simulink model "TrajectoryGenerator3DOF"  (R2023b)
settings: Solver=FixedStepDiscrete  StartTime=0.0  StopTime=1.364*1.4  FixedStep=0.002  RelTol=1e-3
undefined symbols (not defined in the file or in its folder): M_z, Smoothers, Ts
(part 3 of 4)

== system TrajectoryGenerator3DOF/Trajectory Generator17/M22 ==
  x : Inport
  Discrete FIR Filter1 : DiscreteFir  Coefficients=1/N/Ts*[1 zeros(1,N-1) -1]  InitialStates=Q0  SampleTime=Ts
  Discrete Filter : DiscreteFilter  Numerator=[0 Ts]  Denominator=[1 -1]  InitialStates=Q0  SampleTime=Ts
  y : Outport
  dy : Outport  Port=2
  wires:
  Discrete FIR Filter1/1 -> Discrete Filter/1, dy/1
  x/1 -> Discrete FIR Filter1/1
  Discrete Filter/1 -> y/1

== system TrajectoryGenerator3DOF/Trajectory Generator17/M23 ==
  x : Inport
  Discrete FIR Filter1 : DiscreteFir  Coefficients=1/N/Ts*[1 zeros(1,N-1) -1]  InitialStates=Q0  SampleTime=Ts
  Discrete Filter : DiscreteFilter  Numerator=[0 Ts]  Denominator=[1 -1]  InitialStates=Q0  SampleTime=Ts
  y : Outport
  dy : Outport  Port=2
  wires:
  Discrete FIR Filter1/1 -> Discrete Filter/1, dy/1
  x/1 -> Discrete FIR Filter1/1
  Discrete Filter/1 -> y/1

== system TrajectoryGenerator3DOF/Trajectory Generator17/M24 ==
  x : Inport
  Discrete FIR Filter1 : DiscreteFir  Coefficients=1/N/Ts*[1 zeros(1,N-1) -1]  InitialStates=Q0  SampleTime=Ts
  Discrete Filter : DiscreteFilter  Numerator=[0 Ts]  Denominator=[1 -1]  InitialStates=Q0  SampleTime=Ts
  y : Outport
  dy : Outport  Port=2
  wires:
  Discrete FIR Filter1/1 -> Discrete Filter/1, dy/1
  x/1 -> Discrete FIR Filter1/1
  Discrete Filter/1 -> y/1

== system TrajectoryGenerator3DOF/Trajectory Generator17/M33 ==
  x : Inport
  Discrete FIR Filter1 : DiscreteFir  Coefficients=1/N/Ts*[1 zeros(1,N-1) -1]  InitialStates=Q0  SampleTime=Ts
  Discrete Filter : DiscreteFilter  Numerator=[0 Ts]  Denominator=[1 -1]  InitialStates=Q0  SampleTime=Ts
  y : Outport
  dy : Outport  Port=2
  wires:
  Discrete FIR Filter1/1 -> Discrete Filter/1, dy/1
  x/1 -> Discrete FIR Filter1/1
  Discrete Filter/1 -> y/1

== system TrajectoryGenerator3DOF/Trajectory Generator17/M34 ==
  x : Inport
  Discrete FIR Filter1 : DiscreteFir  Coefficients=1/N/Ts*[1 zeros(1,N-1) -1]  InitialStates=Q0  SampleTime=Ts
  Discrete Filter : DiscreteFilter  Numerator=[0 Ts]  Denominator=[1 -1]  InitialStates=Q0  SampleTime=Ts
  y : Outport
  dy : Outport  Port=2
  wires:
  Discrete FIR Filter1/1 -> Discrete Filter/1, dy/1
  x/1 -> Discrete FIR Filter1/1
  Discrete Filter/1 -> y/1

== system TrajectoryGenerator3DOF/Trajectory Generator17/M44 ==
  x : Inport
  Discrete FIR Filter1 : DiscreteFir  Coefficients=1/N/Ts*[1 zeros(1,N-1) -1]  InitialStates=Q0  SampleTime=Ts
  Discrete Filter : DiscreteFilter  Numerator=[0 Ts]  Denominator=[1 -1]  InitialStates=Q0  SampleTime=Ts
  y : Outport
  dy : Outport  Port=2
  wires:
  Discrete FIR Filter1/1 -> Discrete Filter/1, dy/1
  x/1 -> Discrete FIR Filter1/1
  Discrete Filter/1 -> y/1

== system TrajectoryGenerator3DOF/Trajectory Generator18/M11 ==
  x : Inport
  Discrete FIR Filter1 : DiscreteFir  Coefficients=1/N/Ts*[1 zeros(1,N-1) -1]  InitialStates=Q0  SampleTime=Ts
  Discrete Filter : DiscreteFilter  Numerator=[0 Ts]  Denominator=[1 -1]  InitialStates=Q0  SampleTime=Ts
  y : Outport
  dy : Outport  Port=2
  wires:
  Discrete FIR Filter1/1 -> Discrete Filter/1, dy/1
  x/1 -> Discrete FIR Filter1/1
  Discrete Filter/1 -> y/1

== system TrajectoryGenerator3DOF/Trajectory Generator18/M12 ==
  x : Inport
  Discrete FIR Filter1 : DiscreteFir  Coefficients=1/N/Ts*[1 zeros(1,N-1) -1]  InitialStates=Q0  SampleTime=Ts
  Discrete Filter : DiscreteFilter  Numerator=[0 Ts]  Denominator=[1 -1]  InitialStates=Q0  SampleTime=Ts
  y : Outport
  dy : Outport  Port=2
  wires:
  Discrete FIR Filter1/1 -> Discrete Filter/1, dy/1
  x/1 -> Discrete FIR Filter1/1
  Discrete Filter/1 -> y/1

== system TrajectoryGenerator3DOF/Trajectory Generator18/M13 ==
  x : Inport
  Discrete FIR Filter1 : DiscreteFir  Coefficients=1/N/Ts*[1 zeros(1,N-1) -1]  InitialStates=Q0  SampleTime=Ts
  Discrete Filter : DiscreteFilter  Numerator=[0 Ts]  Denominator=[1 -1]  InitialStates=Q0  SampleTime=Ts
  y : Outport
  dy : Outport  Port=2
  wires:
  Discrete FIR Filter1/1 -> Discrete Filter/1, dy/1
  x/1 -> Discrete FIR Filter1/1
  Discrete Filter/1 -> y/1

== system TrajectoryGenerator3DOF/Trajectory Generator18/M14 ==
  x : Inport
  Discrete FIR Filter1 : DiscreteFir  Coefficients=1/N/Ts*[1 zeros(1,N-1) -1]  InitialStates=Q0  SampleTime=Ts
  Discrete Filter : DiscreteFilter  Numerator=[0 Ts]  Denominator=[1 -1]  InitialStates=Q0  SampleTime=Ts
  y : Outport
  dy : Outport  Port=2
  wires:
  Discrete FIR Filter1/1 -> Discrete Filter/1, dy/1
  x/1 -> Discrete FIR Filter1/1
  Discrete Filter/1 -> y/1

== system TrajectoryGenerator3DOF/Trajectory Generator18/M22 ==
  x : Inport
  Discrete FIR Filter1 : DiscreteFir  Coefficients=1/N/Ts*[1 zeros(1,N-1) -1]  InitialStates=Q0  SampleTime=Ts
  Discrete Filter : DiscreteFilter  Numerator=[0 Ts]  Denominator=[1 -1]  InitialStates=Q0  SampleTime=Ts
  y : Outport
  dy : Outport  Port=2
  wires:
  Discrete FIR Filter1/1 -> Discrete Filter/1, dy/1
  x/1 -> Discrete FIR Filter1/1
  Discrete Filter/1 -> y/1

== system TrajectoryGenerator3DOF/Trajectory Generator18/M23 ==
  x : Inport
  Discrete FIR Filter1 : DiscreteFir  Coefficients=1/N/Ts*[1 zeros(1,N-1) -1]  InitialStates=Q0  SampleTime=Ts
  Discrete Filter : DiscreteFilter  Numerator=[0 Ts]  Denominator=[1 -1]  InitialStates=Q0  SampleTime=Ts
  y : Outport
  dy : Outport  Port=2
  wires:
  Discrete FIR Filter1/1 -> Discrete Filter/1, dy/1
  x/1 -> Discrete FIR Filter1/1
  Discrete Filter/1 -> y/1

== system TrajectoryGenerator3DOF/Trajectory Generator18/M24 ==
  x : Inport
  Discrete FIR Filter1 : DiscreteFir  Coefficients=1/N/Ts*[1 zeros(1,N-1) -1]  InitialStates=Q0  SampleTime=Ts
  Discrete Filter : DiscreteFilter  Numerator=[0 Ts]  Denominator=[1 -1]  InitialStates=Q0  SampleTime=Ts
  y : Outport
  dy : Outport  Port=2
  wires:
  Discrete FIR Filter1/1 -> Discrete Filter/1, dy/1
  x/1 -> Discrete FIR Filter1/1
  Discrete Filter/1 -> y/1

== system TrajectoryGenerator3DOF/Trajectory Generator18/M33 ==
  x : Inport
  Discrete FIR Filter1 : DiscreteFir  Coefficients=1/N/Ts*[1 zeros(1,N-1) -1]  InitialStates=Q0  SampleTime=Ts
  Discrete Filter : DiscreteFilter  Numerator=[0 Ts]  Denominator=[1 -1]  InitialStates=Q0  SampleTime=Ts
  y : Outport
  dy : Outport  Port=2
  wires:
  Discrete FIR Filter1/1 -> Discrete Filter/1, dy/1
  x/1 -> Discrete FIR Filter1/1
  Discrete Filter/1 -> y/1

== system TrajectoryGenerator3DOF/Trajectory Generator18/M34 ==
  x : Inport
  Discrete FIR Filter1 : DiscreteFir  Coefficients=1/N/Ts*[1 zeros(1,N-1) -1]  InitialStates=Q0  SampleTime=Ts
  Discrete Filter : DiscreteFilter  Numerator=[0 Ts]  Denominator=[1 -1]  InitialStates=Q0  SampleTime=Ts
  y : Outport
  dy : Outport  Port=2
  wires:
  Discrete FIR Filter1/1 -> Discrete Filter/1, dy/1
  x/1 -> Discrete FIR Filter1/1
  Discrete Filter/1 -> y/1

== system TrajectoryGenerator3DOF/Trajectory Generator18/M44 ==
  x : Inport
  Discrete FIR Filter1 : DiscreteFir  Coefficients=1/N/Ts*[1 zeros(1,N-1) -1]  InitialStates=Q0  SampleTime=Ts
  Discrete Filter : DiscreteFilter  Numerator=[0 Ts]  Denominator=[1 -1]  InitialStates=Q0  SampleTime=Ts
  y : Outport
  dy : Outport  Port=2
  wires:
  Discrete FIR Filter1/1 -> Discrete Filter/1, dy/1
  x/1 -> Discrete FIR Filter1/1
  Discrete Filter/1 -> y/1

== system TrajectoryGenerator3DOF/Trajectory Generator19/M11 ==
  x : Inport
  Discrete FIR Filter1 : DiscreteFir  Coefficients=1/N/Ts*[1 zeros(1,N-1) -1]  InitialStates=Q0  SampleTime=Ts
  Discrete Filter : DiscreteFilter  Numerator=[0 Ts]  Denominator=[1 -1]  InitialStates=Q0  SampleTime=Ts
  y : Outport
  dy : Outport  Port=2
  wires:
  Discrete FIR Filter1/1 -> Discrete Filter/1, dy/1
  x/1 -> Discrete FIR Filter1/1
  Discrete Filter/1 -> y/1

== system TrajectoryGenerator3DOF/Trajectory Generator19/M12 ==
  x : Inport
  Discrete FIR Filter1 : DiscreteFir  Coefficients=1/N/Ts*[1 zeros(1,N-1) -1]  InitialStates=Q0  SampleTime=Ts
  Discrete Filter : DiscreteFilter  Numerator=[0 Ts]  Denominator=[1 -1]  InitialStates=Q0  SampleTime=Ts
  y : Outport
  dy : Outport  Port=2
  wires:
  Discrete FIR Filter1/1 -> Discrete Filter/1, dy/1
  x/1 -> Discrete FIR Filter1/1
  Discrete Filter/1 -> y/1

== system TrajectoryGenerator3DOF/Trajectory Generator19/M13 ==
  x : Inport
  Discrete FIR Filter1 : DiscreteFir  Coefficients=1/N/Ts*[1 zeros(1,N-1) -1]  InitialStates=Q0  SampleTime=Ts
  Discrete Filter : DiscreteFilter  Numerator=[0 Ts]  Denominator=[1 -1]  InitialStates=Q0  SampleTime=Ts
  y : Outport
  dy : Outport  Port=2
  wires:
  Discrete FIR Filter1/1 -> Discrete Filter/1, dy/1
  x/1 -> Discrete FIR Filter1/1
  Discrete Filter/1 -> y/1

== system TrajectoryGenerator3DOF/Trajectory Generator19/M14 ==
  x : Inport
  Discrete FIR Filter1 : DiscreteFir  Coefficients=1/N/Ts*[1 zeros(1,N-1) -1]  InitialStates=Q0  SampleTime=Ts
  Discrete Filter : DiscreteFilter  Numerator=[0 Ts]  Denominator=[1 -1]  InitialStates=Q0  SampleTime=Ts
  y : Outport
  dy : Outport  Port=2
  wires:
  Discrete FIR Filter1/1 -> Discrete Filter/1, dy/1
  x/1 -> Discrete FIR Filter1/1
  Discrete Filter/1 -> y/1

== system TrajectoryGenerator3DOF/Trajectory Generator19/M22 ==
  x : Inport
  Discrete FIR Filter1 : DiscreteFir  Coefficients=1/N/Ts*[1 zeros(1,N-1) -1]  InitialStates=Q0  SampleTime=Ts
  Discrete Filter : DiscreteFilter  Numerator=[0 Ts]  Denominator=[1 -1]  InitialStates=Q0  SampleTime=Ts
  y : Outport
  dy : Outport  Port=2
  wires:
  Discrete FIR Filter1/1 -> Discrete Filter/1, dy/1
  x/1 -> Discrete FIR Filter1/1
  Discrete Filter/1 -> y/1

== system TrajectoryGenerator3DOF/Trajectory Generator19/M23 ==
  x : Inport
  Discrete FIR Filter1 : DiscreteFir  Coefficients=1/N/Ts*[1 zeros(1,N-1) -1]  InitialStates=Q0  SampleTime=Ts
  Discrete Filter : DiscreteFilter  Numerator=[0 Ts]  Denominator=[1 -1]  InitialStates=Q0  SampleTime=Ts
  y : Outport
  dy : Outport  Port=2
  wires:
  Discrete FIR Filter1/1 -> Discrete Filter/1, dy/1
  x/1 -> Discrete FIR Filter1/1
  Discrete Filter/1 -> y/1

== system TrajectoryGenerator3DOF/Trajectory Generator19/M24 ==
  x : Inport
  Discrete FIR Filter1 : DiscreteFir  Coefficients=1/N/Ts*[1 zeros(1,N-1) -1]  InitialStates=Q0  SampleTime=Ts
  Discrete Filter : DiscreteFilter  Numerator=[0 Ts]  Denominator=[1 -1]  InitialStates=Q0  SampleTime=Ts
  y : Outport
  dy : Outport  Port=2
  wires:
  Discrete FIR Filter1/1 -> Discrete Filter/1, dy/1
  x/1 -> Discrete FIR Filter1/1
  Discrete Filter/1 -> y/1

== system TrajectoryGenerator3DOF/Trajectory Generator19/M33 ==
  x : Inport
  Discrete FIR Filter1 : DiscreteFir  Coefficients=1/N/Ts*[1 zeros(1,N-1) -1]  InitialStates=Q0  SampleTime=Ts
  Discrete Filter : DiscreteFilter  Numerator=[0 Ts]  Denominator=[1 -1]  InitialStates=Q0  SampleTime=Ts
  y : Outport
  dy : Outport  Port=2
  wires:
  Discrete FIR Filter1/1 -> Discrete Filter/1, dy/1
  x/1 -> Discrete FIR Filter1/1
  Discrete Filter/1 -> y/1

== system TrajectoryGenerator3DOF/Trajectory Generator19/M34 ==
  x : Inport
  Discrete FIR Filter1 : DiscreteFir  Coefficients=1/N/Ts*[1 zeros(1,N-1) -1]  InitialStates=Q0  SampleTime=Ts
  Discrete Filter : DiscreteFilter  Numerator=[0 Ts]  Denominator=[1 -1]  InitialStates=Q0  SampleTime=Ts
  y : Outport
  dy : Outport  Port=2
  wires:
  Discrete FIR Filter1/1 -> Discrete Filter/1, dy/1
  x/1 -> Discrete FIR Filter1/1
  Discrete Filter/1 -> y/1

== system TrajectoryGenerator3DOF/Trajectory Generator19/M44 ==
  x : Inport
  Discrete FIR Filter1 : DiscreteFir  Coefficients=1/N/Ts*[1 zeros(1,N-1) -1]  InitialStates=Q0  SampleTime=Ts
  Discrete Filter : DiscreteFilter  Numerator=[0 Ts]  Denominator=[1 -1]  InitialStates=Q0  SampleTime=Ts
  y : Outport
  dy : Outport  Port=2
  wires:
  Discrete FIR Filter1/1 -> Discrete Filter/1, dy/1
  x/1 -> Discrete FIR Filter1/1
  Discrete Filter/1 -> y/1

== system TrajectoryGenerator3DOF/Trajectory Generator2/M11 ==
  x : Inport
  Discrete FIR Filter1 : DiscreteFir  Coefficients=1/N/Ts*[1 zeros(1,N-1) -1]  InitialStates=Q0  SampleTime=Ts
  Discrete Filter : DiscreteFilter  Numerator=[0 Ts]  Denominator=[1 -1]  InitialStates=Q0  SampleTime=Ts
  y : Outport
  dy : Outport  Port=2
  wires:
  Discrete FIR Filter1/1 -> Discrete Filter/1, dy/1
  x/1 -> Discrete FIR Filter1/1
  Discrete Filter/1 -> y/1

== system TrajectoryGenerator3DOF/Trajectory Generator2/M12 ==
  x : Inport
  Discrete FIR Filter1 : DiscreteFir  Coefficients=1/N/Ts*[1 zeros(1,N-1) -1]  InitialStates=Q0  SampleTime=Ts
  Discrete Filter : DiscreteFilter  Numerator=[0 Ts]  Denominator=[1 -1]  InitialStates=Q0  SampleTime=Ts
  y : Outport
  dy : Outport  Port=2
  wires:
  Discrete FIR Filter1/1 -> Discrete Filter/1, dy/1
  x/1 -> Discrete FIR Filter1/1
  Discrete Filter/1 -> y/1

== system TrajectoryGenerator3DOF/Trajectory Generator2/M13 ==
  x : Inport
  Discrete FIR Filter1 : DiscreteFir  Coefficients=1/N/Ts*[1 zeros(1,N-1) -1]  InitialStates=Q0  SampleTime=Ts
  Discrete Filter : DiscreteFilter  Numerator=[0 Ts]  Denominator=[1 -1]  InitialStates=Q0  SampleTime=Ts
  y : Outport
  dy : Outport  Port=2
  wires:
  Discrete FIR Filter1/1 -> Discrete Filter/1, dy/1
  x/1 -> Discrete FIR Filter1/1
  Discrete Filter/1 -> y/1

== system TrajectoryGenerator3DOF/Trajectory Generator2/M14 ==
  x : Inport
  Discrete FIR Filter1 : DiscreteFir  Coefficients=1/N/Ts*[1 zeros(1,N-1) -1]  InitialStates=Q0  SampleTime=Ts
  Discrete Filter : DiscreteFilter  Numerator=[0 Ts]  Denominator=[1 -1]  InitialStates=Q0  SampleTime=Ts
  y : Outport
  dy : Outport  Port=2
  wires:
  Discrete FIR Filter1/1 -> Discrete Filter/1, dy/1
  x/1 -> Discrete FIR Filter1/1
  Discrete Filter/1 -> y/1

== system TrajectoryGenerator3DOF/Trajectory Generator2/M22 ==
  x : Inport
  Discrete FIR Filter1 : DiscreteFir  Coefficients=1/N/Ts*[1 zeros(1,N-1) -1]  InitialStates=Q0  SampleTime=Ts
  Discrete Filter : DiscreteFilter  Numerator=[0 Ts]  Denominator=[1 -1]  InitialStates=Q0  SampleTime=Ts
  y : Outport
  dy : Outport  Port=2
  wires:
  Discrete FIR Filter1/1 -> Discrete Filter/1, dy/1
  x/1 -> Discrete FIR Filter1/1
  Discrete Filter/1 -> y/1

== system TrajectoryGenerator3DOF/Trajectory Generator2/M23 ==
  x : Inport
  Discrete FIR Filter1 : DiscreteFir  Coefficients=1/N/Ts*[1 zeros(1,N-1) -1]  InitialStates=Q0  SampleTime=Ts
  Discrete Filter : DiscreteFilter  Numerator=[0 Ts]  Denominator=[1 -1]  InitialStates=Q0  SampleTime=Ts
  y : Outport
  dy : Outport  Port=2
  wires:
  Discrete FIR Filter1/1 -> Discrete Filter/1, dy/1
  x/1 -> Discrete FIR Filter1/1
  Discrete Filter/1 -> y/1

== system TrajectoryGenerator3DOF/Trajectory Generator2/M24 ==
  x : Inport
  Discrete FIR Filter1 : DiscreteFir  Coefficients=1/N/Ts*[1 zeros(1,N-1) -1]  InitialStates=Q0  SampleTime=Ts
  Discrete Filter : DiscreteFilter  Numerator=[0 Ts]  Denominator=[1 -1]  InitialStates=Q0  SampleTime=Ts
  y : Outport
  dy : Outport  Port=2
  wires:
  Discrete FIR Filter1/1 -> Discrete Filter/1, dy/1
  x/1 -> Discrete FIR Filter1/1
  Discrete Filter/1 -> y/1

== system TrajectoryGenerator3DOF/Trajectory Generator2/M33 ==
  x : Inport
  Discrete FIR Filter1 : DiscreteFir  Coefficients=1/N/Ts*[1 zeros(1,N-1) -1]  InitialStates=Q0  SampleTime=Ts
  Discrete Filter : DiscreteFilter  Numerator=[0 Ts]  Denominator=[1 -1]  InitialStates=Q0  SampleTime=Ts
  y : Outport
  dy : Outport  Port=2
  wires:
  Discrete FIR Filter1/1 -> Discrete Filter/1, dy/1
  x/1 -> Discrete FIR Filter1/1
  Discrete Filter/1 -> y/1

== system TrajectoryGenerator3DOF/Trajectory Generator2/M34 ==
  x : Inport
  Discrete FIR Filter1 : DiscreteFir  Coefficients=1/N/Ts*[1 zeros(1,N-1) -1]  InitialStates=Q0  SampleTime=Ts
  Discrete Filter : DiscreteFilter  Numerator=[0 Ts]  Denominator=[1 -1]  InitialStates=Q0  SampleTime=Ts
  y : Outport
  dy : Outport  Port=2
  wires:
  Discrete FIR Filter1/1 -> Discrete Filter/1, dy/1
  x/1 -> Discrete FIR Filter1/1
  Discrete Filter/1 -> y/1

== system TrajectoryGenerator3DOF/Trajectory Generator2/M44 ==
  x : Inport
  Discrete FIR Filter1 : DiscreteFir  Coefficients=1/N/Ts*[1 zeros(1,N-1) -1]  InitialStates=Q0  SampleTime=Ts
  Discrete Filter : DiscreteFilter  Numerator=[0 Ts]  Denominator=[1 -1]  InitialStates=Q0  SampleTime=Ts
  y : Outport
  dy : Outport  Port=2
  wires:
  Discrete FIR Filter1/1 -> Discrete Filter/1, dy/1
  x/1 -> Discrete FIR Filter1/1
  Discrete Filter/1 -> y/1

== system TrajectoryGenerator3DOF/Trajectory Generator20/M11 ==
  x : Inport
  Discrete FIR Filter1 : DiscreteFir  Coefficients=1/N/Ts*[1 zeros(1,N-1) -1]  InitialStates=Q0  SampleTime=Ts
  Discrete Filter : DiscreteFilter  Numerator=[0 Ts]  Denominator=[1 -1]  InitialStates=Q0  SampleTime=Ts
  y : Outport
  dy : Outport  Port=2
  wires:
  Discrete FIR Filter1/1 -> Discrete Filter/1, dy/1
  x/1 -> Discrete FIR Filter1/1
  Discrete Filter/1 -> y/1

== system TrajectoryGenerator3DOF/Trajectory Generator20/M12 ==
  x : Inport
  Discrete FIR Filter1 : DiscreteFir  Coefficients=1/N/Ts*[1 zeros(1,N-1) -1]  InitialStates=Q0  SampleTime=Ts
  Discrete Filter : DiscreteFilter  Numerator=[0 Ts]  Denominator=[1 -1]  InitialStates=Q0  SampleTime=Ts
  y : Outport
  dy : Outport  Port=2
  wires:
  Discrete FIR Filter1/1 -> Discrete Filter/1, dy/1
  x/1 -> Discrete FIR Filter1/1
  Discrete Filter/1 -> y/1

== system TrajectoryGenerator3DOF/Trajectory Generator20/M13 ==
  x : Inport
  Discrete FIR Filter1 : DiscreteFir  Coefficients=1/N/Ts*[1 zeros(1,N-1) -1]  InitialStates=Q0  SampleTime=Ts
  Discrete Filter : DiscreteFilter  Numerator=[0 Ts]  Denominator=[1 -1]  InitialStates=Q0  SampleTime=Ts
  y : Outport
  dy : Outport  Port=2
  wires:
  Discrete FIR Filter1/1 -> Discrete Filter/1, dy/1
  x/1 -> Discrete FIR Filter1/1
  Discrete Filter/1 -> y/1

== system TrajectoryGenerator3DOF/Trajectory Generator20/M14 ==
  x : Inport
  Discrete FIR Filter1 : DiscreteFir  Coefficients=1/N/Ts*[1 zeros(1,N-1) -1]  InitialStates=Q0  SampleTime=Ts
  Discrete Filter : DiscreteFilter  Numerator=[0 Ts]  Denominator=[1 -1]  InitialStates=Q0  SampleTime=Ts
  y : Outport
  dy : Outport  Port=2
  wires:
  Discrete FIR Filter1/1 -> Discrete Filter/1, dy/1
  x/1 -> Discrete FIR Filter1/1
  Discrete Filter/1 -> y/1

== system TrajectoryGenerator3DOF/Trajectory Generator20/M22 ==
  x : Inport
  Discrete FIR Filter1 : DiscreteFir  Coefficients=1/N/Ts*[1 zeros(1,N-1) -1]  InitialStates=Q0  SampleTime=Ts
  Discrete Filter : DiscreteFilter  Numerator=[0 Ts]  Denominator=[1 -1]  InitialStates=Q0  SampleTime=Ts
  y : Outport
  dy : Outport  Port=2
  wires:
  Discrete FIR Filter1/1 -> Discrete Filter/1, dy/1
  x/1 -> Discrete FIR Filter1/1
  Discrete Filter/1 -> y/1

== system TrajectoryGenerator3DOF/Trajectory Generator20/M23 ==
  x : Inport
  Discrete FIR Filter1 : DiscreteFir  Coefficients=1/N/Ts*[1 zeros(1,N-1) -1]  InitialStates=Q0  SampleTime=Ts
  Discrete Filter : DiscreteFilter  Numerator=[0 Ts]  Denominator=[1 -1]  InitialStates=Q0  SampleTime=Ts
  y : Outport
  dy : Outport  Port=2
  wires:
  Discrete FIR Filter1/1 -> Discrete Filter/1, dy/1
  x/1 -> Discrete FIR Filter1/1
  Discrete Filter/1 -> y/1

== system TrajectoryGenerator3DOF/Trajectory Generator20/M24 ==
  x : Inport
  Discrete FIR Filter1 : DiscreteFir  Coefficients=1/N/Ts*[1 zeros(1,N-1) -1]  InitialStates=Q0  SampleTime=Ts
  Discrete Filter : DiscreteFilter  Numerator=[0 Ts]  Denominator=[1 -1]  InitialStates=Q0  SampleTime=Ts
  y : Outport
  dy : Outport  Port=2
  wires:
  Discrete FIR Filter1/1 -> Discrete Filter/1, dy/1
  x/1 -> Discrete FIR Filter1/1
  Discrete Filter/1 -> y/1

== system TrajectoryGenerator3DOF/Trajectory Generator20/M33 ==
  x : Inport
  Discrete FIR Filter1 : DiscreteFir  Coefficients=1/N/Ts*[1 zeros(1,N-1) -1]  InitialStates=Q0  SampleTime=Ts
  Discrete Filter : DiscreteFilter  Numerator=[0 Ts]  Denominator=[1 -1]  InitialStates=Q0  SampleTime=Ts
  y : Outport
  dy : Outport  Port=2
  wires:
  Discrete FIR Filter1/1 -> Discrete Filter/1, dy/1
  x/1 -> Discrete FIR Filter1/1
  Discrete Filter/1 -> y/1

== system TrajectoryGenerator3DOF/Trajectory Generator20/M34 ==
  x : Inport
  Discrete FIR Filter1 : DiscreteFir  Coefficients=1/N/Ts*[1 zeros(1,N-1) -1]  InitialStates=Q0  SampleTime=Ts
  Discrete Filter : DiscreteFilter  Numerator=[0 Ts]  Denominator=[1 -1]  InitialStates=Q0  SampleTime=Ts
  y : Outport
  dy : Outport  Port=2
  wires:
  Discrete FIR Filter1/1 -> Discrete Filter/1, dy/1
  x/1 -> Discrete FIR Filter1/1
  Discrete Filter/1 -> y/1

== system TrajectoryGenerator3DOF/Trajectory Generator20/M44 ==
  x : Inport
  Discrete FIR Filter1 : DiscreteFir  Coefficients=1/N/Ts*[1 zeros(1,N-1) -1]  InitialStates=Q0  SampleTime=Ts
  Discrete Filter : DiscreteFilter  Numerator=[0 Ts]  Denominator=[1 -1]  InitialStates=Q0  SampleTime=Ts
  y : Outport
  dy : Outport  Port=2
  wires:
  Discrete FIR Filter1/1 -> Discrete Filter/1, dy/1
  x/1 -> Discrete FIR Filter1/1
  Discrete Filter/1 -> y/1

== system TrajectoryGenerator3DOF/Trajectory Generator21/M11 ==
  x : Inport
  Discrete FIR Filter1 : DiscreteFir  Coefficients=1/N/Ts*[1 zeros(1,N-1) -1]  InitialStates=Q0  SampleTime=Ts
  Discrete Filter : DiscreteFilter  Numerator=[0 Ts]  Denominator=[1 -1]  InitialStates=Q0  SampleTime=Ts
  y : Outport
  dy : Outport  Port=2
  wires:
  Discrete FIR Filter1/1 -> Discrete Filter/1, dy/1
  x/1 -> Discrete FIR Filter1/1
  Discrete Filter/1 -> y/1

== system TrajectoryGenerator3DOF/Trajectory Generator21/M12 ==
  x : Inport
  Discrete FIR Filter1 : DiscreteFir  Coefficients=1/N/Ts*[1 zeros(1,N-1) -1]  InitialStates=Q0  SampleTime=Ts
  Discrete Filter : DiscreteFilter  Numerator=[0 Ts]  Denominator=[1 -1]  InitialStates=Q0  SampleTime=Ts
  y : Outport
  dy : Outport  Port=2
  wires:
  Discrete FIR Filter1/1 -> Discrete Filter/1, dy/1
  x/1 -> Discrete FIR Filter1/1
  Discrete Filter/1 -> y/1

== system TrajectoryGenerator3DOF/Trajectory Generator21/M13 ==
  x : Inport
  Discrete FIR Filter1 : DiscreteFir  Coefficients=1/N/Ts*[1 zeros(1,N-1) -1]  InitialStates=Q0  SampleTime=Ts
  Discrete Filter : DiscreteFilter  Numerator=[0 Ts]  Denominator=[1 -1]  InitialStates=Q0  SampleTime=Ts
  y : Outport
  dy : Outport  Port=2
  wires:
  Discrete FIR Filter1/1 -> Discrete Filter/1, dy/1
  x/1 -> Discrete FIR Filter1/1
  Discrete Filter/1 -> y/1

== system TrajectoryGenerator3DOF/Trajectory Generator21/M14 ==
  x : Inport
  Discrete FIR Filter1 : DiscreteFir  Coefficients=1/N/Ts*[1 zeros(1,N-1) -1]  InitialStates=Q0  SampleTime=Ts
  Discrete Filter : DiscreteFilter  Numerator=[0 Ts]  Denominator=[1 -1]  InitialStates=Q0  SampleTime=Ts
  y : Outport
  dy : Outport  Port=2
  wires:
  Discrete FIR Filter1/1 -> Discrete Filter/1, dy/1
  x/1 -> Discrete FIR Filter1/1
  Discrete Filter/1 -> y/1

== system TrajectoryGenerator3DOF/Trajectory Generator21/M22 ==
  x : Inport
  Discrete FIR Filter1 : DiscreteFir  Coefficients=1/N/Ts*[1 zeros(1,N-1) -1]  InitialStates=Q0  SampleTime=Ts
  Discrete Filter : DiscreteFilter  Numerator=[0 Ts]  Denominator=[1 -1]  InitialStates=Q0  SampleTime=Ts
  y : Outport
  dy : Outport  Port=2
  wires:
  Discrete FIR Filter1/1 -> Discrete Filter/1, dy/1
  x/1 -> Discrete FIR Filter1/1
  Discrete Filter/1 -> y/1

== system TrajectoryGenerator3DOF/Trajectory Generator21/M23 ==
  x : Inport
  Discrete FIR Filter1 : DiscreteFir  Coefficients=1/N/Ts*[1 zeros(1,N-1) -1]  InitialStates=Q0  SampleTime=Ts
  Discrete Filter : DiscreteFilter  Numerator=[0 Ts]  Denominator=[1 -1]  InitialStates=Q0  SampleTime=Ts
  y : Outport
  dy : Outport  Port=2
  wires:
  Discrete FIR Filter1/1 -> Discrete Filter/1, dy/1
  x/1 -> Discrete FIR Filter1/1
  Discrete Filter/1 -> y/1

== system TrajectoryGenerator3DOF/Trajectory Generator21/M24 ==
  x : Inport
  Discrete FIR Filter1 : DiscreteFir  Coefficients=1/N/Ts*[1 zeros(1,N-1) -1]  InitialStates=Q0  SampleTime=Ts
  Discrete Filter : DiscreteFilter  Numerator=[0 Ts]  Denominator=[1 -1]  InitialStates=Q0  SampleTime=Ts
  y : Outport
  dy : Outport  Port=2
  wires:
  Discrete FIR Filter1/1 -> Discrete Filter/1, dy/1
  x/1 -> Discrete FIR Filter1/1
  Discrete Filter/1 -> y/1

== system TrajectoryGenerator3DOF/Trajectory Generator21/M33 ==
  x : Inport
  Discrete FIR Filter1 : DiscreteFir  Coefficients=1/N/Ts*[1 zeros(1,N-1) -1]  InitialStates=Q0  SampleTime=Ts
  Discrete Filter : DiscreteFilter  Numerator=[0 Ts]  Denominator=[1 -1]  InitialStates=Q0  SampleTime=Ts
  y : Outport
  dy : Outport  Port=2
  wires:
  Discrete FIR Filter1/1 -> Discrete Filter/1, dy/1
  x/1 -> Discrete FIR Filter1/1
  Discrete Filter/1 -> y/1

== system TrajectoryGenerator3DOF/Trajectory Generator21/M34 ==
  x : Inport
  Discrete FIR Filter1 : DiscreteFir  Coefficients=1/N/Ts*[1 zeros(1,N-1) -1]  InitialStates=Q0  SampleTime=Ts
  Discrete Filter : DiscreteFilter  Numerator=[0 Ts]  Denominator=[1 -1]  InitialStates=Q0  SampleTime=Ts
  y : Outport
  dy : Outport  Port=2
  wires:
  Discrete FIR Filter1/1 -> Discrete Filter/1, dy/1
  x/1 -> Discrete FIR Filter1/1
  Discrete Filter/1 -> y/1

== system TrajectoryGenerator3DOF/Trajectory Generator21/M44 ==
  x : Inport
  Discrete FIR Filter1 : DiscreteFir  Coefficients=1/N/Ts*[1 zeros(1,N-1) -1]  InitialStates=Q0  SampleTime=Ts
  Discrete Filter : DiscreteFilter  Numerator=[0 Ts]  Denominator=[1 -1]  InitialStates=Q0  SampleTime=Ts
  y : Outport
  dy : Outport  Port=2
  wires:
  Discrete FIR Filter1/1 -> Discrete Filter/1, dy/1
  x/1 -> Discrete FIR Filter1/1
  Discrete Filter/1 -> y/1

== system TrajectoryGenerator3DOF/Trajectory Generator3/M11 ==
  x : Inport
  Discrete FIR Filter1 : DiscreteFir  Coefficients=1/N/Ts*[1 zeros(1,N-1) -1]  InitialStates=Q0  SampleTime=Ts
  Discrete Filter : DiscreteFilter  Numerator=[0 Ts]  Denominator=[1 -1]  InitialStates=Q0  SampleTime=Ts
  y : Outport
  dy : Outport  Port=2
  wires:
  Discrete FIR Filter1/1 -> Discrete Filter/1, dy/1
  x/1 -> Discrete FIR Filter1/1
  Discrete Filter/1 -> y/1

== system TrajectoryGenerator3DOF/Trajectory Generator3/M12 ==
  x : Inport
  Discrete FIR Filter1 : DiscreteFir  Coefficients=1/N/Ts*[1 zeros(1,N-1) -1]  InitialStates=Q0  SampleTime=Ts
  Discrete Filter : DiscreteFilter  Numerator=[0 Ts]  Denominator=[1 -1]  InitialStates=Q0  SampleTime=Ts
  y : Outport
  dy : Outport  Port=2
  wires:
  Discrete FIR Filter1/1 -> Discrete Filter/1, dy/1
  x/1 -> Discrete FIR Filter1/1
  Discrete Filter/1 -> y/1

== system TrajectoryGenerator3DOF/Trajectory Generator3/M13 ==
  x : Inport
  Discrete FIR Filter1 : DiscreteFir  Coefficients=1/N/Ts*[1 zeros(1,N-1) -1]  InitialStates=Q0  SampleTime=Ts
  Discrete Filter : DiscreteFilter  Numerator=[0 Ts]  Denominator=[1 -1]  InitialStates=Q0  SampleTime=Ts
  y : Outport
  dy : Outport  Port=2
  wires:
  Discrete FIR Filter1/1 -> Discrete Filter/1, dy/1
  x/1 -> Discrete FIR Filter1/1
  Discrete Filter/1 -> y/1

== system TrajectoryGenerator3DOF/Trajectory Generator3/M14 ==
  x : Inport
  Discrete FIR Filter1 : DiscreteFir  Coefficients=1/N/Ts*[1 zeros(1,N-1) -1]  InitialStates=Q0  SampleTime=Ts
  Discrete Filter : DiscreteFilter  Numerator=[0 Ts]  Denominator=[1 -1]  InitialStates=Q0  SampleTime=Ts
  y : Outport
  dy : Outport  Port=2
  wires:
  Discrete FIR Filter1/1 -> Discrete Filter/1, dy/1
  x/1 -> Discrete FIR Filter1/1
  Discrete Filter/1 -> y/1

== system TrajectoryGenerator3DOF/Trajectory Generator3/M22 ==
  x : Inport
  Discrete FIR Filter1 : DiscreteFir  Coefficients=1/N/Ts*[1 zeros(1,N-1) -1]  InitialStates=Q0  SampleTime=Ts
  Discrete Filter : DiscreteFilter  Numerator=[0 Ts]  Denominator=[1 -1]  InitialStates=Q0  SampleTime=Ts
  y : Outport
  dy : Outport  Port=2
  wires:
  Discrete FIR Filter1/1 -> Discrete Filter/1, dy/1
  x/1 -> Discrete FIR Filter1/1
  Discrete Filter/1 -> y/1

== system TrajectoryGenerator3DOF/Trajectory Generator3/M23 ==
  x : Inport
  Discrete FIR Filter1 : DiscreteFir  Coefficients=1/N/Ts*[1 zeros(1,N-1) -1]  InitialStates=Q0  SampleTime=Ts
  Discrete Filter : DiscreteFilter  Numerator=[0 Ts]  Denominator=[1 -1]  InitialStates=Q0  SampleTime=Ts
  y : Outport
  dy : Outport  Port=2
  wires:
  Discrete FIR Filter1/1 -> Discrete Filter/1, dy/1
  x/1 -> Discrete FIR Filter1/1
  Discrete Filter/1 -> y/1

== system TrajectoryGenerator3DOF/Trajectory Generator3/M24 ==
  x : Inport
  Discrete FIR Filter1 : DiscreteFir  Coefficients=1/N/Ts*[1 zeros(1,N-1) -1]  InitialStates=Q0  SampleTime=Ts
  Discrete Filter : DiscreteFilter  Numerator=[0 Ts]  Denominator=[1 -1]  InitialStates=Q0  SampleTime=Ts
  y : Outport
  dy : Outport  Port=2
  wires:
  Discrete FIR Filter1/1 -> Discrete Filter/1, dy/1
  x/1 -> Discrete FIR Filter1/1
  Discrete Filter/1 -> y/1

== system TrajectoryGenerator3DOF/Trajectory Generator3/M33 ==
  x : Inport
  Discrete FIR Filter1 : DiscreteFir  Coefficients=1/N/Ts*[1 zeros(1,N-1) -1]  InitialStates=Q0  SampleTime=Ts
  Discrete Filter : DiscreteFilter  Numerator=[0 Ts]  Denominator=[1 -1]  InitialStates=Q0  SampleTime=Ts
  y : Outport
  dy : Outport  Port=2
  wires:
  Discrete FIR Filter1/1 -> Discrete Filter/1, dy/1
  x/1 -> Discrete FIR Filter1/1
  Discrete Filter/1 -> y/1

== system TrajectoryGenerator3DOF/Trajectory Generator3/M34 ==
  x : Inport
  Discrete FIR Filter1 : DiscreteFir  Coefficients=1/N/Ts*[1 zeros(1,N-1) -1]  InitialStates=Q0  SampleTime=Ts
  Discrete Filter : DiscreteFilter  Numerator=[0 Ts]  Denominator=[1 -1]  InitialStates=Q0  SampleTime=Ts
  y : Outport
  dy : Outport  Port=2
  wires:
  Discrete FIR Filter1/1 -> Discrete Filter/1, dy/1
  x/1 -> Discrete FIR Filter1/1
  Discrete Filter/1 -> y/1

== system TrajectoryGenerator3DOF/Trajectory Generator3/M44 ==
  x : Inport
  Discrete FIR Filter1 : DiscreteFir  Coefficients=1/N/Ts*[1 zeros(1,N-1) -1]  InitialStates=Q0  SampleTime=Ts
  Discrete Filter : DiscreteFilter  Numerator=[0 Ts]  Denominator=[1 -1]  InitialStates=Q0  SampleTime=Ts
  y : Outport
  dy : Outport  Port=2
  wires:
  Discrete FIR Filter1/1 -> Discrete Filter/1, dy/1
  x/1 -> Discrete FIR Filter1/1
  Discrete Filter/1 -> y/1

== system TrajectoryGenerator3DOF/Trajectory Generator4/M11 ==
  x : Inport
  Discrete FIR Filter1 : DiscreteFir  Coefficients=1/N/Ts*[1 zeros(1,N-1) -1]  InitialStates=Q0  SampleTime=Ts
  Discrete Filter : DiscreteFilter  Numerator=[0 Ts]  Denominator=[1 -1]  InitialStates=Q0  SampleTime=Ts
  y : Outport
  dy : Outport  Port=2
  wires:
  Discrete FIR Filter1/1 -> Discrete Filter/1, dy/1
  x/1 -> Discrete FIR Filter1/1
  Discrete Filter/1 -> y/1

== system TrajectoryGenerator3DOF/Trajectory Generator4/M12 ==
  x : Inport
  Discrete FIR Filter1 : DiscreteFir  Coefficients=1/N/Ts*[1 zeros(1,N-1) -1]  InitialStates=Q0  SampleTime=Ts
  Discrete Filter : DiscreteFilter  Numerator=[0 Ts]  Denominator=[1 -1]  InitialStates=Q0  SampleTime=Ts
  y : Outport
  dy : Outport  Port=2
  wires:
  Discrete FIR Filter1/1 -> Discrete Filter/1, dy/1
  x/1 -> Discrete FIR Filter1/1
  Discrete Filter/1 -> y/1

== system TrajectoryGenerator3DOF/Trajectory Generator4/M13 ==
  x : Inport
  Discrete FIR Filter1 : DiscreteFir  Coefficients=1/N/Ts*[1 zeros(1,N-1) -1]  InitialStates=Q0  SampleTime=Ts
  Discrete Filter : DiscreteFilter  Numerator=[0 Ts]  Denominator=[1 -1]  InitialStates=Q0  SampleTime=Ts
  y : Outport
  dy : Outport  Port=2
  wires:
  Discrete FIR Filter1/1 -> Discrete Filter/1, dy/1
  x/1 -> Discrete FIR Filter1/1
  Discrete Filter/1 -> y/1

== system TrajectoryGenerator3DOF/Trajectory Generator4/M14 ==
  x : Inport
  Discrete FIR Filter1 : DiscreteFir  Coefficients=1/N/Ts*[1 zeros(1,N-1) -1]  InitialStates=Q0  SampleTime=Ts
  Discrete Filter : DiscreteFilter  Numerator=[0 Ts]  Denominator=[1 -1]  InitialStates=Q0  SampleTime=Ts
  y : Outport
  dy : Outport  Port=2
  wires:
  Discrete FIR Filter1/1 -> Discrete Filter/1, dy/1
  x/1 -> Discrete FIR Filter1/1
  Discrete Filter/1 -> y/1

== system TrajectoryGenerator3DOF/Trajectory Generator4/M22 ==
  x : Inport
  Discrete FIR Filter1 : DiscreteFir  Coefficients=1/N/Ts*[1 zeros(1,N-1) -1]  InitialStates=Q0  SampleTime=Ts
  Discrete Filter : DiscreteFilter  Numerator=[0 Ts]  Denominator=[1 -1]  InitialStates=Q0  SampleTime=Ts
  y : Outport
  dy : Outport  Port=2
  wires:
  Discrete FIR Filter1/1 -> Discrete Filter/1, dy/1
  x/1 -> Discrete FIR Filter1/1
  Discrete Filter/1 -> y/1

== system TrajectoryGenerator3DOF/Trajectory Generator4/M23 ==
  x : Inport
  Discrete FIR Filter1 : DiscreteFir  Coefficients=1/N/Ts*[1 zeros(1,N-1) -1]  InitialStates=Q0  SampleTime=Ts
  Discrete Filter : DiscreteFilter  Numerator=[0 Ts]  Denominator=[1 -1]  InitialStates=Q0  SampleTime=Ts
  y : Outport
  dy : Outport  Port=2
  wires:
  Discrete FIR Filter1/1 -> Discrete Filter/1, dy/1
  x/1 -> Discrete FIR Filter1/1
  Discrete Filter/1 -> y/1

== system TrajectoryGenerator3DOF/Trajectory Generator4/M24 ==
  x : Inport
  Discrete FIR Filter1 : DiscreteFir  Coefficients=1/N/Ts*[1 zeros(1,N-1) -1]  InitialStates=Q0  SampleTime=Ts
  Discrete Filter : DiscreteFilter  Numerator=[0 Ts]  Denominator=[1 -1]  InitialStates=Q0  SampleTime=Ts
  y : Outport
  dy : Outport  Port=2
  wires:
  Discrete FIR Filter1/1 -> Discrete Filter/1, dy/1
  x/1 -> Discrete FIR Filter1/1
  Discrete Filter/1 -> y/1

== system TrajectoryGenerator3DOF/Trajectory Generator4/M33 ==
  x : Inport
  Discrete FIR Filter1 : DiscreteFir  Coefficients=1/N/Ts*[1 zeros(1,N-1) -1]  InitialStates=Q0  SampleTime=Ts
  Discrete Filter : DiscreteFilter  Numerator=[0 Ts]  Denominator=[1 -1]  InitialStates=Q0  SampleTime=Ts
  y : Outport
  dy : Outport  Port=2
  wires:
  Discrete FIR Filter1/1 -> Discrete Filter/1, dy/1
  x/1 -> Discrete FIR Filter1/1
  Discrete Filter/1 -> y/1

== system TrajectoryGenerator3DOF/Trajectory Generator4/M34 ==
  x : Inport
  Discrete FIR Filter1 : DiscreteFir  Coefficients=1/N/Ts*[1 zeros(1,N-1) -1]  InitialStates=Q0  SampleTime=Ts
  Discrete Filter : DiscreteFilter  Numerator=[0 Ts]  Denominator=[1 -1]  InitialStates=Q0  SampleTime=Ts
  y : Outport
  dy : Outport  Port=2
  wires:
  Discrete FIR Filter1/1 -> Discrete Filter/1, dy/1
  x/1 -> Discrete FIR Filter1/1
  Discrete Filter/1 -> y/1

== system TrajectoryGenerator3DOF/Trajectory Generator4/M44 ==
  x : Inport
  Discrete FIR Filter1 : DiscreteFir  Coefficients=1/N/Ts*[1 zeros(1,N-1) -1]  InitialStates=Q0  SampleTime=Ts
  Discrete Filter : DiscreteFilter  Numerator=[0 Ts]  Denominator=[1 -1]  InitialStates=Q0  SampleTime=Ts
  y : Outport
  dy : Outport  Port=2
  wires:
  Discrete FIR Filter1/1 -> Discrete Filter/1, dy/1
  x/1 -> Discrete FIR Filter1/1
  Discrete Filter/1 -> y/1

== system TrajectoryGenerator3DOF/Trajectory Generator5/M11 ==
  x : Inport
  Discrete FIR Filter1 : DiscreteFir  Coefficients=1/N/Ts*[1 zeros(1,N-1) -1]  InitialStates=Q0  SampleTime=Ts
  Discrete Filter : DiscreteFilter  Numerator=[0 Ts]  Denominator=[1 -1]  InitialStates=Q0  SampleTime=Ts
  y : Outport
  dy : Outport  Port=2
  wires:
  Discrete FIR Filter1/1 -> Discrete Filter/1, dy/1
  x/1 -> Discrete FIR Filter1/1
  Discrete Filter/1 -> y/1

== system TrajectoryGenerator3DOF/Trajectory Generator5/M12 ==
  x : Inport
  Discrete FIR Filter1 : DiscreteFir  Coefficients=1/N/Ts*[1 zeros(1,N-1) -1]  InitialStates=Q0  SampleTime=Ts
  Discrete Filter : DiscreteFilter  Numerator=[0 Ts]  Denominator=[1 -1]  InitialStates=Q0  SampleTime=Ts
  y : Outport
  dy : Outport  Port=2
  wires:
  Discrete FIR Filter1/1 -> Discrete Filter/1, dy/1
  x/1 -> Discrete FIR Filter1/1
  Discrete Filter/1 -> y/1

== system TrajectoryGenerator3DOF/Trajectory Generator5/M13 ==
  x : Inport
  Discrete FIR Filter1 : DiscreteFir  Coefficients=1/N/Ts*[1 zeros(1,N-1) -1]  InitialStates=Q0  SampleTime=Ts
  Discrete Filter : DiscreteFilter  Numerator=[0 Ts]  Denominator=[1 -1]  InitialStates=Q0  SampleTime=Ts
  y : Outport
  dy : Outport  Port=2
  wires:
  Discrete FIR Filter1/1 -> Discrete Filter/1, dy/1
  x/1 -> Discrete FIR Filter1/1
  Discrete Filter/1 -> y/1

== system TrajectoryGenerator3DOF/Trajectory Generator5/M14 ==
  x : Inport
  Discrete FIR Filter1 : DiscreteFir  Coefficients=1/N/Ts*[1 zeros(1,N-1) -1]  InitialStates=Q0  SampleTime=Ts
  Discrete Filter : DiscreteFilter  Numerator=[0 Ts]  Denominator=[1 -1]  InitialStates=Q0  SampleTime=Ts
  y : Outport
  dy : Outport  Port=2
  wires:
  Discrete FIR Filter1/1 -> Discrete Filter/1, dy/1
  x/1 -> Discrete FIR Filter1/1
  Discrete Filter/1 -> y/1

== system TrajectoryGenerator3DOF/Trajectory Generator5/M22 ==
  x : Inport
  Discrete FIR Filter1 : DiscreteFir  Coefficients=1/N/Ts*[1 zeros(1,N-1) -1]  InitialStates=Q0  SampleTime=Ts
  Discrete Filter : DiscreteFilter  Numerator=[0 Ts]  Denominator=[1 -1]  InitialStates=Q0  SampleTime=Ts
  y : Outport
  dy : Outport  Port=2
  wires:
  Discrete FIR Filter1/1 -> Discrete Filter/1, dy/1
  x/1 -> Discrete FIR Filter1/1
  Discrete Filter/1 -> y/1

== system TrajectoryGenerator3DOF/Trajectory Generator5/M23 ==
  x : Inport
  Discrete FIR Filter1 : DiscreteFir  Coefficients=1/N/Ts*[1 zeros(1,N-1) -1]  InitialStates=Q0  SampleTime=Ts
  Discrete Filter : DiscreteFilter  Numerator=[0 Ts]  Denominator=[1 -1]  InitialStates=Q0  SampleTime=Ts
  y : Outport
  dy : Outport  Port=2
  wires:
  Discrete FIR Filter1/1 -> Discrete Filter/1, dy/1
  x/1 -> Discrete FIR Filter1/1
  Discrete Filter/1 -> y/1

== system TrajectoryGenerator3DOF/Trajectory Generator5/M24 ==
  x : Inport
  Discrete FIR Filter1 : DiscreteFir  Coefficients=1/N/Ts*[1 zeros(1,N-1) -1]  InitialStates=Q0  SampleTime=Ts
  Discrete Filter : DiscreteFilter  Numerator=[0 Ts]  Denominator=[1 -1]  InitialStates=Q0  SampleTime=Ts
  y : Outport
  dy : Outport  Port=2
  wires:
  Discrete FIR Filter1/1 -> Discrete Filter/1, dy/1
  x/1 -> Discrete FIR Filter1/1
  Discrete Filter/1 -> y/1

== system TrajectoryGenerator3DOF/Trajectory Generator5/M33 ==
  x : Inport
  Discrete FIR Filter1 : DiscreteFir  Coefficients=1/N/Ts*[1 zeros(1,N-1) -1]  InitialStates=Q0  SampleTime=Ts
  Discrete Filter : DiscreteFilter  Numerator=[0 Ts]  Denominator=[1 -1]  InitialStates=Q0  SampleTime=Ts
  y : Outport
  dy : Outport  Port=2
  wires:
  Discrete FIR Filter1/1 -> Discrete Filter/1, dy/1
  x/1 -> Discrete FIR Filter1/1
  Discrete Filter/1 -> y/1

== system TrajectoryGenerator3DOF/Trajectory Generator5/M34 ==
  x : Inport
  Discrete FIR Filter1 : DiscreteFir  Coefficients=1/N/Ts*[1 zeros(1,N-1) -1]  InitialStates=Q0  SampleTime=Ts
  Discrete Filter : DiscreteFilter  Numerator=[0 Ts]  Denominator=[1 -1]  InitialStates=Q0  SampleTime=Ts
  y : Outport
  dy : Outport  Port=2
  wires:
  Discrete FIR Filter1/1 -> Discrete Filter/1, dy/1
  x/1 -> Discrete FIR Filter1/1
  Discrete Filter/1 -> y/1

== system TrajectoryGenerator3DOF/Trajectory Generator5/M44 ==
  x : Inport
  Discrete FIR Filter1 : DiscreteFir  Coefficients=1/N/Ts*[1 zeros(1,N-1) -1]  InitialStates=Q0  SampleTime=Ts
  Discrete Filter : DiscreteFilter  Numerator=[0 Ts]  Denominator=[1 -1]  InitialStates=Q0  SampleTime=Ts
  y : Outport
  dy : Outport  Port=2
  wires:
  Discrete FIR Filter1/1 -> Discrete Filter/1, dy/1
  x/1 -> Discrete FIR Filter1/1
  Discrete Filter/1 -> y/1

== system TrajectoryGenerator3DOF/Trajectory Generator6/M11 ==
  x : Inport
  Discrete FIR Filter1 : DiscreteFir  Coefficients=1/N/Ts*[1 zeros(1,N-1) -1]  InitialStates=Q0  SampleTime=Ts
  Discrete Filter : DiscreteFilter  Numerator=[0 Ts]  Denominator=[1 -1]  InitialStates=Q0  SampleTime=Ts
  y : Outport
  dy : Outport  Port=2
  wires:
  Discrete FIR Filter1/1 -> Discrete Filter/1, dy/1
  x/1 -> Discrete FIR Filter1/1
  Discrete Filter/1 -> y/1

== system TrajectoryGenerator3DOF/Trajectory Generator6/M12 ==
  x : Inport
  Discrete FIR Filter1 : DiscreteFir  Coefficients=1/N/Ts*[1 zeros(1,N-1) -1]  InitialStates=Q0  SampleTime=Ts
  Discrete Filter : DiscreteFilter  Numerator=[0 Ts]  Denominator=[1 -1]  InitialStates=Q0  SampleTime=Ts
  y : Outport
  dy : Outport  Port=2
  wires:
  Discrete FIR Filter1/1 -> Discrete Filter/1, dy/1
  x/1 -> Discrete FIR Filter1/1
  Discrete Filter/1 -> y/1

== system TrajectoryGenerator3DOF/Trajectory Generator6/M13 ==
  x : Inport
  Discrete FIR Filter1 : DiscreteFir  Coefficients=1/N/Ts*[1 zeros(1,N-1) -1]  InitialStates=Q0  SampleTime=Ts
  Discrete Filter : DiscreteFilter  Numerator=[0 Ts]  Denominator=[1 -1]  InitialStates=Q0  SampleTime=Ts
  y : Outport
  dy : Outport  Port=2
  wires:
  Discrete FIR Filter1/1 -> Discrete Filter/1, dy/1
  x/1 -> Discrete FIR Filter1/1
  Discrete Filter/1 -> y/1

== system TrajectoryGenerator3DOF/Trajectory Generator6/M14 ==
  x : Inport
  Discrete FIR Filter1 : DiscreteFir  Coefficients=1/N/Ts*[1 zeros(1,N-1) -1]  InitialStates=Q0  SampleTime=Ts
  Discrete Filter : DiscreteFilter  Numerator=[0 Ts]  Denominator=[1 -1]  InitialStates=Q0  SampleTime=Ts
  y : Outport
  dy : Outport  Port=2
  wires:
  Discrete FIR Filter1/1 -> Discrete Filter/1, dy/1
  x/1 -> Discrete FIR Filter1/1
  Discrete Filter/1 -> y/1

== system TrajectoryGenerator3DOF/Trajectory Generator6/M22 ==
  x : Inport
  Discrete FIR Filter1 : DiscreteFir  Coefficients=1/N/Ts*[1 zeros(1,N-1) -1]  InitialStates=Q0  SampleTime=Ts
  Discrete Filter : DiscreteFilter  Numerator=[0 Ts]  Denominator=[1 -1]  InitialStates=Q0  SampleTime=Ts
  y : Outport
  dy : Outport  Port=2
  wires:
  Discrete FIR Filter1/1 -> Discrete Filter/1, dy/1
  x/1 -> Discrete FIR Filter1/1
  Discrete Filter/1 -> y/1

== system TrajectoryGenerator3DOF/Trajectory Generator6/M23 ==
  x : Inport
  Discrete FIR Filter1 : DiscreteFir  Coefficients=1/N/Ts*[1 zeros(1,N-1) -1]  InitialStates=Q0  SampleTime=Ts
  Discrete Filter : DiscreteFilter  Numerator=[0 Ts]  Denominator=[1 -1]  InitialStates=Q0  SampleTime=Ts
  y : Outport
  dy : Outport  Port=2
  wires:
  Discrete FIR Filter1/1 -> Discrete Filter/1, dy/1
  x/1 -> Discrete FIR Filter1/1
  Discrete Filter/1 -> y/1

== system TrajectoryGenerator3DOF/Trajectory Generator6/M24 ==
  x : Inport
  Discrete FIR Filter1 : DiscreteFir  Coefficients=1/N/Ts*[1 zeros(1,N-1) -1]  InitialStates=Q0  SampleTime=Ts
  Discrete Filter : DiscreteFilter  Numerator=[0 Ts]  Denominator=[1 -1]  InitialStates=Q0  SampleTime=Ts
  y : Outport
  dy : Outport  Port=2
  wires:
  Discrete FIR Filter1/1 -> Discrete Filter/1, dy/1
  x/1 -> Discrete FIR Filter1/1
  Discrete Filter/1 -> y/1

== system TrajectoryGenerator3DOF/Trajectory Generator6/M33 ==
  x : Inport
  Discrete FIR Filter1 : DiscreteFir  Coefficients=1/N/Ts*[1 zeros(1,N-1) -1]  InitialStates=Q0  SampleTime=Ts
  Discrete Filter : DiscreteFilter  Numerator=[0 Ts]  Denominator=[1 -1]  InitialStates=Q0  SampleTime=Ts
  y : Outport
  dy : Outport  Port=2
  wires:
  Discrete FIR Filter1/1 -> Discrete Filter/1, dy/1
  x/1 -> Discrete FIR Filter1/1
  Discrete Filter/1 -> y/1

== system TrajectoryGenerator3DOF/Trajectory Generator6/M34 ==
  x : Inport
  Discrete FIR Filter1 : DiscreteFir  Coefficients=1/N/Ts*[1 zeros(1,N-1) -1]  InitialStates=Q0  SampleTime=Ts
  Discrete Filter : DiscreteFilter  Numerator=[0 Ts]  Denominator=[1 -1]  InitialStates=Q0  SampleTime=Ts
  y : Outport
  dy : Outport  Port=2
  wires:
  Discrete FIR Filter1/1 -> Discrete Filter/1, dy/1
  x/1 -> Discrete FIR Filter1/1
  Discrete Filter/1 -> y/1

== system TrajectoryGenerator3DOF/Trajectory Generator6/M44 ==
  x : Inport
  Discrete FIR Filter1 : DiscreteFir  Coefficients=1/N/Ts*[1 zeros(1,N-1) -1]  InitialStates=Q0  SampleTime=Ts
  Discrete Filter : DiscreteFilter  Numerator=[0 Ts]  Denominator=[1 -1]  InitialStates=Q0  SampleTime=Ts
  y : Outport
  dy : Outport  Port=2
  wires:
  Discrete FIR Filter1/1 -> Discrete Filter/1, dy/1
  x/1 -> Discrete FIR Filter1/1
  Discrete Filter/1 -> y/1

== system TrajectoryGenerator3DOF/Trajectory Generator7/M11 ==
  x : Inport
  Discrete FIR Filter1 : DiscreteFir  Coefficients=1/N/Ts*[1 zeros(1,N-1) -1]  InitialStates=Q0  SampleTime=Ts
  Discrete Filter : DiscreteFilter  Numerator=[0 Ts]  Denominator=[1 -1]  InitialStates=Q0  SampleTime=Ts
  y : Outport
  dy : Outport  Port=2
  wires:
  Discrete FIR Filter1/1 -> Discrete Filter/1, dy/1
  x/1 -> Discrete FIR Filter1/1
  Discrete Filter/1 -> y/1

== system TrajectoryGenerator3DOF/Trajectory Generator7/M12 ==
  x : Inport
  Discrete FIR Filter1 : DiscreteFir  Coefficients=1/N/Ts*[1 zeros(1,N-1) -1]  InitialStates=Q0  SampleTime=Ts
  Discrete Filter : DiscreteFilter  Numerator=[0 Ts]  Denominator=[1 -1]  InitialStates=Q0  SampleTime=Ts
  y : Outport
  dy : Outport  Port=2
  wires:
  Discrete FIR Filter1/1 -> Discrete Filter/1, dy/1
  x/1 -> Discrete FIR Filter1/1
  Discrete Filter/1 -> y/1

== system TrajectoryGenerator3DOF/Trajectory Generator7/M13 ==
  x : Inport
  Discrete FIR Filter1 : DiscreteFir  Coefficients=1/N/Ts*[1 zeros(1,N-1) -1]  InitialStates=Q0  SampleTime=Ts
  Discrete Filter : DiscreteFilter  Numerator=[0 Ts]  Denominator=[1 -1]  InitialStates=Q0  SampleTime=Ts
  y : Outport
  dy : Outport  Port=2
  wires:
  Discrete FIR Filter1/1 -> Discrete Filter/1, dy/1
  x/1 -> Discrete FIR Filter1/1
  Discrete Filter/1 -> y/1

== system TrajectoryGenerator3DOF/Trajectory Generator7/M14 ==
  x : Inport
  Discrete FIR Filter1 : DiscreteFir  Coefficients=1/N/Ts*[1 zeros(1,N-1) -1]  InitialStates=Q0  SampleTime=Ts
  Discrete Filter : DiscreteFilter  Numerator=[0 Ts]  Denominator=[1 -1]  InitialStates=Q0  SampleTime=Ts
  y : Outport
  dy : Outport  Port=2
  wires:
  Discrete FIR Filter1/1 -> Discrete Filter/1, dy/1
  x/1 -> Discrete FIR Filter1/1
  Discrete Filter/1 -> y/1

== system TrajectoryGenerator3DOF/Trajectory Generator7/M22 ==
  x : Inport
  Discrete FIR Filter1 : DiscreteFir  Coefficients=1/N/Ts*[1 zeros(1,N-1) -1]  InitialStates=Q0  SampleTime=Ts
  Discrete Filter : DiscreteFilter  Numerator=[0 Ts]  Denominator=[1 -1]  InitialStates=Q0  SampleTime=Ts
  y : Outport
  dy : Outport  Port=2
  wires:
  Discrete FIR Filter1/1 -> Discrete Filter/1, dy/1
  x/1 -> Discrete FIR Filter1/1
  Discrete Filter/1 -> y/1

== system TrajectoryGenerator3DOF/Trajectory Generator7/M23 ==
  x : Inport
  Discrete FIR Filter1 : DiscreteFir  Coefficients=1/N/Ts*[1 zeros(1,N-1) -1]  InitialStates=Q0  SampleTime=Ts
  Discrete Filter : DiscreteFilter  Numerator=[0 Ts]  Denominator=[1 -1]  InitialStates=Q0  SampleTime=Ts
  y : Outport
  dy : Outport  Port=2
  wires:
  Discrete FIR Filter1/1 -> Discrete Filter/1, dy/1
  x/1 -> Discrete FIR Filter1/1
  Discrete Filter/1 -> y/1

== system TrajectoryGenerator3DOF/Trajectory Generator7/M24 ==
  x : Inport
  Discrete FIR Filter1 : DiscreteFir  Coefficients=1/N/Ts*[1 zeros(1,N-1) -1]  InitialStates=Q0  SampleTime=Ts
  Discrete Filter : DiscreteFilter  Numerator=[0 Ts]  Denominator=[1 -1]  InitialStates=Q0  SampleTime=Ts
  y : Outport
  dy : Outport  Port=2
  wires:
  Discrete FIR Filter1/1 -> Discrete Filter/1, dy/1
  x/1 -> Discrete FIR Filter1/1
  Discrete Filter/1 -> y/1

== system TrajectoryGenerator3DOF/Trajectory Generator7/M33 ==
  x : Inport
  Discrete FIR Filter1 : DiscreteFir  Coefficients=1/N/Ts*[1 zeros(1,N-1) -1]  InitialStates=Q0  SampleTime=Ts
  Discrete Filter : DiscreteFilter  Numerator=[0 Ts]  Denominator=[1 -1]  InitialStates=Q0  SampleTime=Ts
  y : Outport
  dy : Outport  Port=2
  wires:
  Discrete FIR Filter1/1 -> Discrete Filter/1, dy/1
  x/1 -> Discrete FIR Filter1/1
  Discrete Filter/1 -> y/1

== system TrajectoryGenerator3DOF/Trajectory Generator7/M34 ==
  x : Inport
  Discrete FIR Filter1 : DiscreteFir  Coefficients=1/N/Ts*[1 zeros(1,N-1) -1]  InitialStates=Q0  SampleTime=Ts
  Discrete Filter : DiscreteFilter  Numerator=[0 Ts]  Denominator=[1 -1]  InitialStates=Q0  SampleTime=Ts
  y : Outport
  dy : Outport  Port=2
  wires:
  Discrete FIR Filter1/1 -> Discrete Filter/1, dy/1
  x/1 -> Discrete FIR Filter1/1
  Discrete Filter/1 -> y/1

== system TrajectoryGenerator3DOF/Trajectory Generator7/M44 ==
  x : Inport
  Discrete FIR Filter1 : DiscreteFir  Coefficients=1/N/Ts*[1 zeros(1,N-1) -1]  InitialStates=Q0  SampleTime=Ts
  Discrete Filter : DiscreteFilter  Numerator=[0 Ts]  Denominator=[1 -1]  InitialStates=Q0  SampleTime=Ts
  y : Outport
  dy : Outport  Port=2
  wires:
  Discrete FIR Filter1/1 -> Discrete Filter/1, dy/1
  x/1 -> Discrete FIR Filter1/1
  Discrete Filter/1 -> y/1

== system TrajectoryGenerator3DOF/Trajectory Generator8/M11 ==
  x : Inport
  Discrete FIR Filter1 : DiscreteFir  Coefficients=1/N/Ts*[1 zeros(1,N-1) -1]  InitialStates=Q0  SampleTime=Ts
  Discrete Filter : DiscreteFilter  Numerator=[0 Ts]  Denominator=[1 -1]  InitialStates=Q0  SampleTime=Ts
  y : Outport
  dy : Outport  Port=2
  wires:
  Discrete FIR Filter1/1 -> Discrete Filter/1, dy/1
  x/1 -> Discrete FIR Filter1/1
  Discrete Filter/1 -> y/1

== system TrajectoryGenerator3DOF/Trajectory Generator8/M12 ==
  x : Inport
  Discrete FIR Filter1 : DiscreteFir  Coefficients=1/N/Ts*[1 zeros(1,N-1) -1]  InitialStates=Q0  SampleTime=Ts
  Discrete Filter : DiscreteFilter  Numerator=[0 Ts]  Denominator=[1 -1]  InitialStates=Q0  SampleTime=Ts
  y : Outport
  dy : Outport  Port=2
  wires:
  Discrete FIR Filter1/1 -> Discrete Filter/1, dy/1
  x/1 -> Discrete FIR Filter1/1
  Discrete Filter/1 -> y/1

== system TrajectoryGenerator3DOF/Trajectory Generator8/M13 ==
  x : Inport
  Discrete FIR Filter1 : DiscreteFir  Coefficients=1/N/Ts*[1 zeros(1,N-1) -1]  InitialStates=Q0  SampleTime=Ts
  Discrete Filter : DiscreteFilter  Numerator=[0 Ts]  Denominator=[1 -1]  InitialStates=Q0  SampleTime=Ts
  y : Outport
  dy : Outport  Port=2
  wires:
  Discrete FIR Filter1/1 -> Discrete Filter/1, dy/1
  x/1 -> Discrete FIR Filter1/1
  Discrete Filter/1 -> y/1

== system TrajectoryGenerator3DOF/Trajectory Generator8/M14 ==
  x : Inport
  Discrete FIR Filter1 : DiscreteFir  Coefficients=1/N/Ts*[1 zeros(1,N-1) -1]  InitialStates=Q0  SampleTime=Ts
  Discrete Filter : DiscreteFilter  Numerator=[0 Ts]  Denominator=[1 -1]  InitialStates=Q0  SampleTime=Ts
  y : Outport
  dy : Outport  Port=2
  wires:
  Discrete FIR Filter1/1 -> Discrete Filter/1, dy/1
  x/1 -> Discrete FIR Filter1/1
  Discrete Filter/1 -> y/1
